simulink model "pid_motor_control_simulink"  (R2020b)
settings: Solver=VariableStepAuto  StartTime=0.0  StopTime=10.0  RelTol=1e-3
settings Model: Creator=kuzub  LastModifiedBy=kuzub

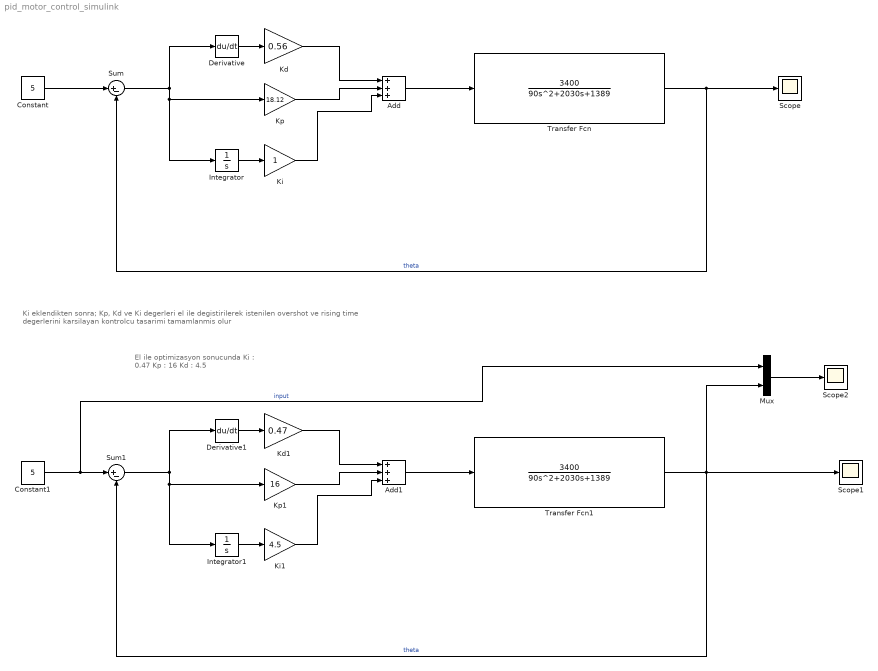
== system pid_motor_control_simulink ==
  note: El ile optimizasyon sonucunda
      | 	Ki  : 0.47
      | 	Kp : 16
      | 	Kd : 4.5
  note: Ki eklendikten sonra; Kp, Kd ve Ki degerleri el ile degistirilerek istenilen overshot ve rising time degerlerini karsilayan kontrolcu tasarimi tamamlanmis olur
  Add : Sum  Inputs=+++
  Add1 : Sum  Inputs=+++
  Constant : Constant  Value=5
  Constant1 : Constant  Value=5
  Derivative : Derivative
  Derivative1 : Derivative
  Integrator : Integrator
  Integrator1 : Integrator
  Kd : Gain  Gain=0.56
  Kd1 : Gain  Gain=0.47
  Ki : Gain
  Ki1 : Gain  Gain=4.5
  Kp : Gain  Gain=18.12
  Kp1 : Gain  Gain=16
  Mux : Mux  Inputs=2
  Scope : Scope
  Scope1 : Scope
  Scope2 : Scope
  Sum : Sum  Inputs=|+-
  Sum1 : Sum  Inputs=|+-
  Transfer Fcn : TransferFcn  Numerator=[3400]  Denominator=[90 2030 1389]
  Transfer Fcn1 : TransferFcn  Numerator=[3400]  Denominator=[90 2030 1389]
  wires:
  Constant/1 -> Sum/1
  Transfer Fcn/1 -> Scope/1, Sum/2  "theta"
  Add/1 -> Transfer Fcn/1
  Kd/1 -> Add/1
  Kp/1 -> Add/2
  Derivative/1 -> Kd/1
  Ki/1 -> Add/3
  Integrator/1 -> Ki/1
  Sum/1 -> Derivative/1, Integrator/1, Kp/1
  Sum1/1 -> Kp1/1, Integrator1/1, Derivative1/1
  Integrator1/1 -> Ki1/1
  Ki1/1 -> Add1/3
  Derivative1/1 -> Kd1/1
  Kp1/1 -> Add1/2
  Kd1/1 -> Add1/1
  Add1/1 -> Transfer Fcn1/1
  Transfer Fcn1/1 -> Mux/2, Sum1/2, Scope1/1  "theta"
  Constant1/1 -> Mux/1, Sum1/1  "input"
  Mux/1 -> Scope2/1
